simulink model "AreaCoverage"  (R2024a)
settings: Solver=FixedStepDiscrete  StartTime=0.0  StopTime=Tf  RelTol=1e-2
undefined symbols (not defined in the file or in its folder): g0, maxsteps, obsMat, s0
libraries: rllib x3
settings Model: Creator=abiswas  LastModifiedBy=chris
settings SolverCC: AlgebraicLoopSolver=TrustRegion
settings DebuggingCC: UnconnectedInputMsg=warning  UnconnectedOutputMsg=warning  UnconnectedLineMsg=warning
settings ModelReferenceCC: EnableRefExpFcnMdlSchedulingChecks=on
settings RTWCC: GPUComputeCapability=3.5  DLArmComputeVersion=19.05

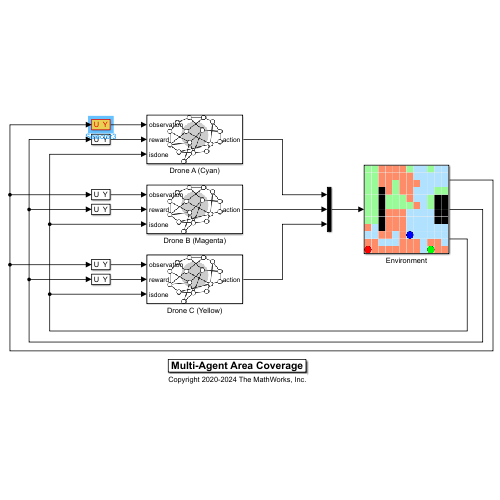
[thumbnail: Simulink's stored preview of the top-level diagram]
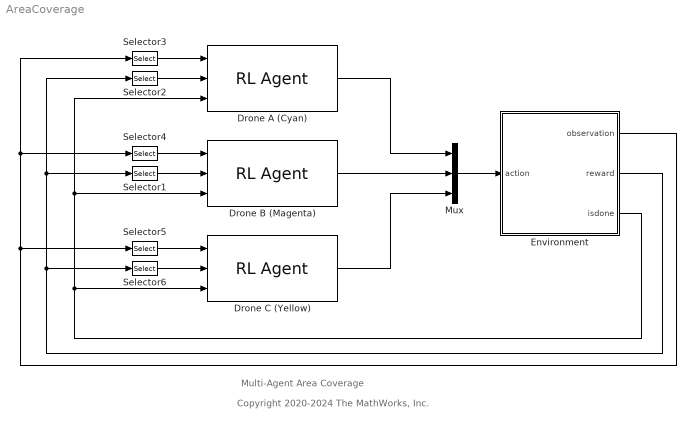
== system AreaCoverage ==
  note: Copyright 2020-2024 The MathWorks, Inc.
  note: Multi-Agent Area Coverage
  Drone A (Cyan) : rllib/RL Agent  Agent=agentA  ExternalActionAsInput=off  ProvideLastAction=off  ProvideCumRwd=off  TreatAsDirectFeedthrough=on  UseStrictObservationDataTypes=off
  Drone B (Magenta) : rllib/RL Agent  Agent=agentB  ExternalActionAsInput=off  ProvideLastAction=off  ProvideCumRwd=off  TreatAsDirectFeedthrough=on  UseStrictObservationDataTypes=off
  Drone C (Yellow) : rllib/RL Agent  Agent=agentC  ExternalActionAsInput=off  ProvideLastAction=off  ProvideCumRwd=off  TreatAsDirectFeedthrough=on  UseStrictObservationDataTypes=off
  Environment : Subsystem
      mask Display: image('area.png');
  Mux : Mux  Inputs=3
  Selector1 : Selector  InputPortWidth=3  IndexOptions=Index vector (dialog)  Indices=2  OutputSizes=1
  Selector2 : Selector  InputPortWidth=3  IndexOptions=Index vector (dialog)  Indices=1  OutputSizes=1
  Selector3 : Selector  NumberOfDimensions=4  InputPortWidth=3  IndexOptions=Select all,Select all,Select all,Index vector (dialog)  Indices=1,1,1,1  OutputSizes=1,1,1,1
  Selector4 : Selector  NumberOfDimensions=4  InputPortWidth=3  IndexOptions=Select all,Select all,Select all,Index vector (dialog)  Indices=1,1,1,2  OutputSizes=1,1,1,1
  Selector5 : Selector  NumberOfDimensions=4  InputPortWidth=3  IndexOptions=Select all,Select all,Select all,Index vector (dialog)  Indices=1,1,1,3  OutputSizes=1,1,1,1
  Selector6 : Selector  InputPortWidth=3  IndexOptions=Index vector (dialog)  Indices=3  OutputSizes=1
  wires:
  Drone B (Magenta)/1 -> Mux/2
  Drone A (Cyan)/1 -> Mux/1
  Selector3/1 -> Drone A (Cyan)/1
  Selector2/1 -> Drone A (Cyan)/2
  Selector1/1 -> Drone B (Magenta)/2
  Selector4/1 -> Drone B (Magenta)/1
  Drone C (Yellow)/1 -> Mux/3
  Selector5/1 -> Drone C (Yellow)/1
  Selector6/1 -> Drone C (Yellow)/2
  Environment/3(isdone) -> Drone B (Magenta)/3, Drone A (Cyan)/3, Drone C (Yellow)/3
  Environment/1(observation) -> Selector3/1, Selector4/1, Selector5/1
  Environment/2(reward) -> Selector2/1, Selector1/1, Selector6/1
  Mux/1 -> Environment/1(action)

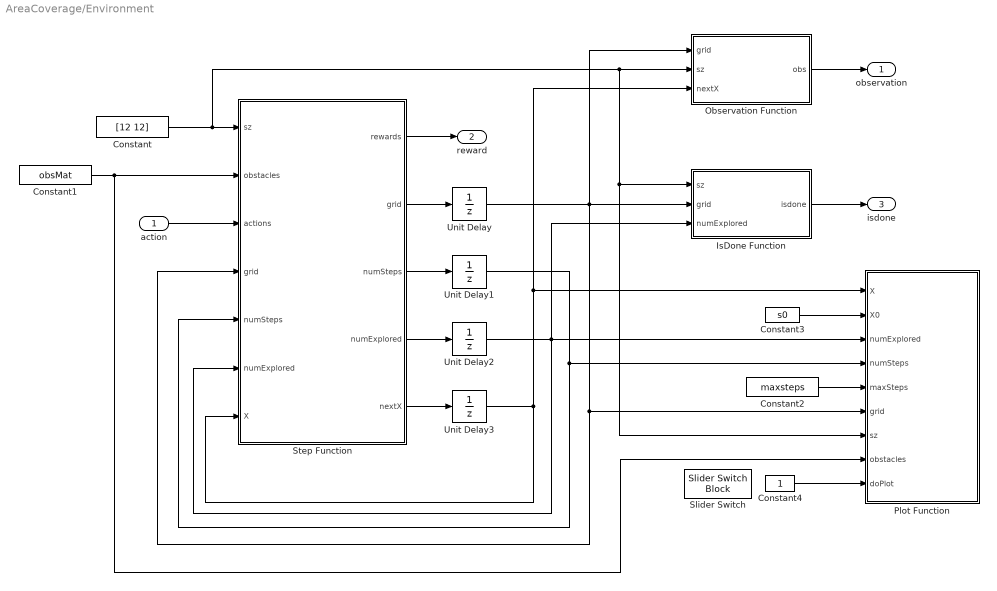
== system AreaCoverage/Environment ==
  action : Inport
  Constant : Constant  Value=[12 12]
  Constant1 : Constant  Value=obsMat
  Constant2 : Constant  Value=maxsteps
  Constant3 : Constant  Value=s0
  Constant4 : Constant
  IsDone Function : MATLAB Function  TreatAsAtomicUnit=on
  Observation Function : MATLAB Function  TreatAsAtomicUnit=on
  Plot Function : MATLAB Function  TreatAsAtomicUnit=on
  Slider Switch : SliderSwitchBlock  LabelPosition=Hide
      settings: Values={{'Off', 'On'}, [0 1]}
  Step Function : MATLAB Function  TreatAsAtomicUnit=on
  Unit Delay : UnitDelay  InitialCondition=g0  SampleTime=-1  HasFrameUpgradeWarning=on
  Unit Delay1 : UnitDelay  SampleTime=-1  HasFrameUpgradeWarning=on
  Unit Delay2 : UnitDelay  InitialCondition=ones(1,3)  SampleTime=-1  HasFrameUpgradeWarning=on
  Unit Delay3 : UnitDelay  InitialCondition=s0  SampleTime=-1  HasFrameUpgradeWarning=on
  observation : Outport
  reward : Outport  Port=2
  isdone : Outport  Port=3
  wires:
  Step Function/2(grid) -> Unit Delay/1
  Observation Function/1(obs) -> observation/1
  Step Function/1(rewards) -> reward/1
  Step Function/3(numSteps) -> Unit Delay1/1
  Step Function/4(numExplored) -> Unit Delay2/1
  Step Function/5(nextX) -> Unit Delay3/1
  IsDone Function/1(isdone) -> isdone/1
  Constant3/1 -> Plot Function/2(X0)
  Constant/1 -> Observation Function/2(sz), Plot Function/7(sz), IsDone Function/1(sz), Step Function/1(sz)
  Constant1/1 -> Step Function/2(obstacles), Plot Function/8(obstacles)
  action/1 -> Step Function/3(actions)
  Unit Delay3/1 -> Step Function/7(X), Observation Function/3(nextX), Plot Function/1(X)
  Unit Delay2/1 -> Step Function/6("numExplored "), Plot Function/3(numExplored), IsDone Function/3(numExplored)
  Unit Delay1/1 -> Step Function/5("numSteps "), Plot Function/4(numSteps)
  Unit Delay/1 -> Observation Function/1(grid), IsDone Function/2(grid), Step Function/4("grid "), Plot Function/6(grid)
  Constant2/1 -> Plot Function/5(maxSteps)
  Constant4/1 -> Plot Function/9(doPlot)

== matlab function AreaCoverage/Environment/Observation Function ==
  data: grid input size=[12,12]; obs output size=[12,12,4,3]; sz input size=[1,2]; nextX input size=[3,2]
function obs = observation(grid,sz,nextX)
% Observation for each agent is a 12x12 4-channel image. The
% channels are:
% 1. Obstacle channel - cells with obstacles are 1, rest 0
% 2. Self channel - cell with the agent's state is 1, rest 0
% 3. Friend channel - cell with other agent's state is 1, rest 0
% 4. Coverage channel - cells that are unexplored are 1, rest 0

% Copyright 2024 The MathWorks, Inc.

obs = zeros(12,12,4,3);
numRobots = 3;

for idx = 1:numRobots
    obstacleChannel = 1 * (grid == 1.0);

    selfIdx = idx;
    selfRow = nextX(selfIdx,1);
    selfCol = nextX(selfIdx,2);
    selfChannel = zeros(sz);
    selfChannel(selfRow,selfCol) = 1;

    friendIdxs = idx ~= (1:numRobots);
    friendRows = nextX(friendIdxs,1);
    friendCols = nextX(friendIdxs,2);
    friendChannel = zeros(sz);
    friendChannel(friendRows(1),friendCols(1)) = 1;
    friendChannel(friendRows(2),friendCols(2)) = 1;

    coverageChannel = 1.0 * (grid == 0);

    obs(:,:,1,idx) = obstacleChannel;
    obs(:,:,2,idx) = selfChannel;
    obs(:,:,3,idx) = friendChannel;
    obs(:,:,4,idx) = coverageChannel;
end

== matlab function AreaCoverage/Environment/Step Function ==
  data: sz input size=[1,2]; obstacles input; actions input; grid input; numSteps input; numExplored input size=[1,3]; rewards output; grid output; numSteps output; numExplored output size=[1,3]; nextX output; X input
function [rewards,grid,numSteps,numExplored,nextX] = stepEnvironment(sz,obstacles,actions,grid,numSteps,numExplored,X)
% Environment step function.
%
% Reward:
%
% Moves to unexplored cell: +2
% Move out of grid/collision: -1
% No movement: -1
% Full coverage: +100

% Copyright 2024 The MathWorks, Inc.

numRobots = 3;

% move robots to their next state
rewards = zeros(numRobots,1);
nextStates = X;
for idx = 1:numRobots
    rbtState = X(idx,:);
    rbtAction = actions(idx);
    switch(rbtAction)
        case 0
            % Wait
            nextStates(idx,:) = rbtState;
            rewards(idx) = rewards(idx) - 1; % lazy penalty
        case 1
            % Move up
            if rbtState(1) < sz(1) && ~checkCollision(obstacles,rbtState+[1 0],nextStates(idx~=1:numRobots,:))
                nextStates(idx,:) = rbtState + [1 0];
            else
                % penalty for collision with obstacle or boundary
                nextStates(idx,:) = rbtState;
                rewards(idx) = rewards(idx) - 1;
            end
        case 2
            % Move down
            if rbtState(1) > 1 && ~checkCollision(obstacles,rbtState+[-1 0],nextStates(idx~=1:numRobots,:))
                nextStates(idx,:) = rbtState + [-1 0];
            else
                % penalty for collision with obstacle or boundary
                nextStates(idx,:) = rbtState;
                rewards(idx) = rewards(idx) - 1;
            end
        case 3
            % Move left
            if rbtState(2) > 1 && ~checkCollision(obstacles,rbtState+[0 -1],nextStates(idx~=1:numRobots,:))
                nextStates(idx,:) = rbtState + [0 -1];
            else
                % penalty for collision with obstacle or boundary
                nextStates(idx,:) = rbtState;
                rewards(idx) = rewards(idx) - 1;
            end
        case 4
            % Move right
            if rbtState(2) < sz(2) && ~checkCollision(obstacles,rbtState+[0 1],nextStates(idx~=1:numRobots,:))
                nextStates(idx,:) = rbtState + [0 1];
            else
                % penalty for collision with obstacle or boundary
                nextStates(idx,:) = rbtState;
                rewards(idx) = rewards(idx) - 1; %rewards(idx) - 10;
            end
    end
end

% update grid and reward agents for new exploration
for idx = 1:numRobots
    r = nextStates(idx,1);
    c = nextStates(idx,2);
    if grid(r,c) == 0.0
        % robot explores an unexplored cell
        rewards(idx) = rewards(idx) + 10;
        % update grid values
        switch(idx)
            case 1
                grid(r,c) = 0.25;  % explored by A
                numExplored = numExplored + [1 0 0];
            case 2
                grid(r,c) = 0.5;   % explored by B
                numExplored = numExplored + [0 1 0];
            case 3
                grid(r,c) = 0.75;   % explored by C
                numExplored = numExplored + [0 0 1];
        end 
    else
        % provide a small penalty for an explored cell
        rewards(idx) = rewards(idx) - 0.5;
    end
end

% coverage metrics
totalExploredCells = sum(numExplored);
totalCells = sz(1) * sz(2) - sum(grid==1,'all');

% full coverage reward
if totalExploredCells >= totalCells
    rewards = rewards + 100;
end

% Update states
nextX = nextStates;
numSteps = numSteps + 1;

end


function collision = checkCollision(obstacles,new_state,other_states)
% Create array of occupied states
if isequal(obstacles,-1)
    occupiedStates = other_states;
else
    occupiedStates = [other_states; obstacles];
end
% check collision
collision = any(all(new_state==occupiedStates,2));
end

== matlab function AreaCoverage/Environment/IsDone Function ==
  data: sz input; isdone output; grid input; numExplored input
function isdone = isDone(sz,grid,numExplored)
% Is Done condition

% Copyright 2024 The MathWorks, Inc.

isdone = 0;
totalExploredCells = sum(numExplored);
totalCells = sz(1) * sz(2) - sum(grid==1,'all');
if totalExploredCells >= totalCells
    isdone = 1;
end

== matlab function AreaCoverage/Environment/Plot Function ==
  data: X input; X0 input; numExplored input; numSteps input; maxSteps input; grid input; sz input; obstacles input; doPlot input
function plotEnv(X,X0,numExplored,numSteps,maxSteps,grid,sz,obstacles,doPlot)
% Plot environment

% Copyright 2024 The MathWorks, Inc.

coder.extrinsic("plotGrid");

if doPlot && numSteps <= maxSteps
    plotGrid(X,X0,numExplored,numSteps,grid,sz,obstacles);
end
